simulink model "Arduino"  (R2023a)
settings: Solver=VariableStepAuto  StartTime=0.0  StopTime=inf  RelTol=1e-3
settings Model: Creator=paragmraw  LastModifiedBy=paragmraw

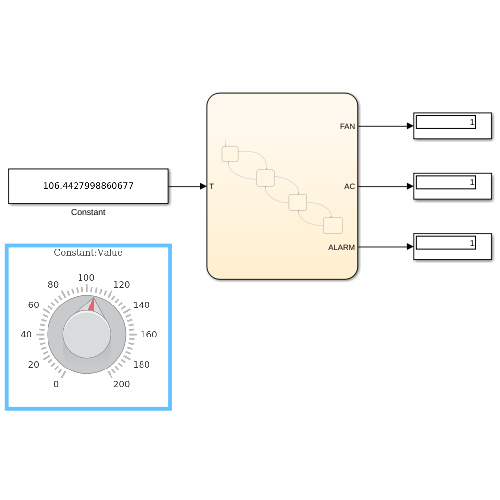
[thumbnail: Simulink's stored preview of the top-level diagram]
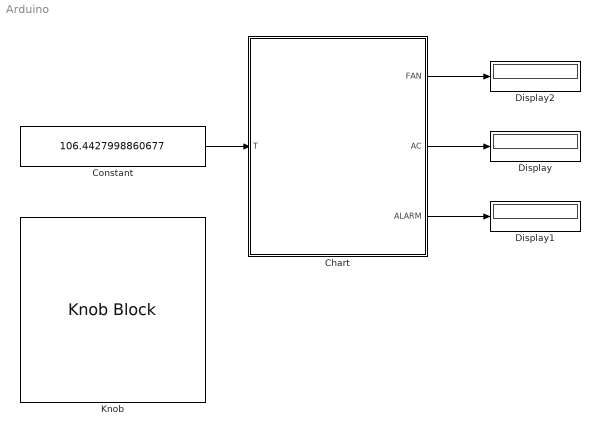
== system Arduino ==
  Chart : Stateflow chart  TreatAsAtomicUnit=on
  Constant : Constant  Value=106.4427998860677  VectorParams1D=off  SampleTime=-1
  Display : Display
  Display1 : Display
  Display2 : Display
  Knob : KnobBlock  ScaleMax=200
  wires:
  Constant/1 -> Chart/1(T)
  Chart/2(AC) -> Display/1
  Chart/3(ALARM) -> Display1/1
  Chart/1(FAN) -> Display2/1

== stateflow chart Arduino/Chart ==
  state OFF_
    entry:
    FAN=0;
    AC=0;
    ALARM=0;
  state FAN_ON
    entry:
    FAN=1;
    AC=0;
    ALARM=0;
  state AC_ON
    entry:
    FAN=1;
    AC=1;
    ALARM=0;
  state ALARM_ON
    entry:
    FAN=1;
    AC=1;
    ALARM=1;
  (default) -> OFF_
  OFF_ -> FAN_ON : [T>=50]
  FAN_ON -> OFF_ [order 2] : [T<50]
  FAN_ON -> AC_ON [order 1] : [T>=70]
  AC_ON -> FAN_ON [order 1] : [T<70]
  AC_ON -> ALARM_ON [order 2] : [T>=90]
  ALARM_ON -> AC_ON : [T<90]
  data: FAN output [0..1]; T input; AC output [0..1]; ALARM output [0..1]
